simulink model "RGP_regression_th"  (R2018b)
settings: Solver=FixedStepAuto  StartTime=0.0  StopTime=timeVec(end)  FixedStep=(timeVec(2)-timeVec(1))  RelTol=1e-3
values from neighbouring files (symbols this model uses):
  postVarCtrlGain = 1    [RGP_regression_ts.m]
libraries: simulink x2, RGP_ctrl x1, RGP_regression x1
settings Model: Creator=asiddiq2  LastModifiedBy=Ayaz
settings DataIOCC: ReturnWorkspaceOutputs=on

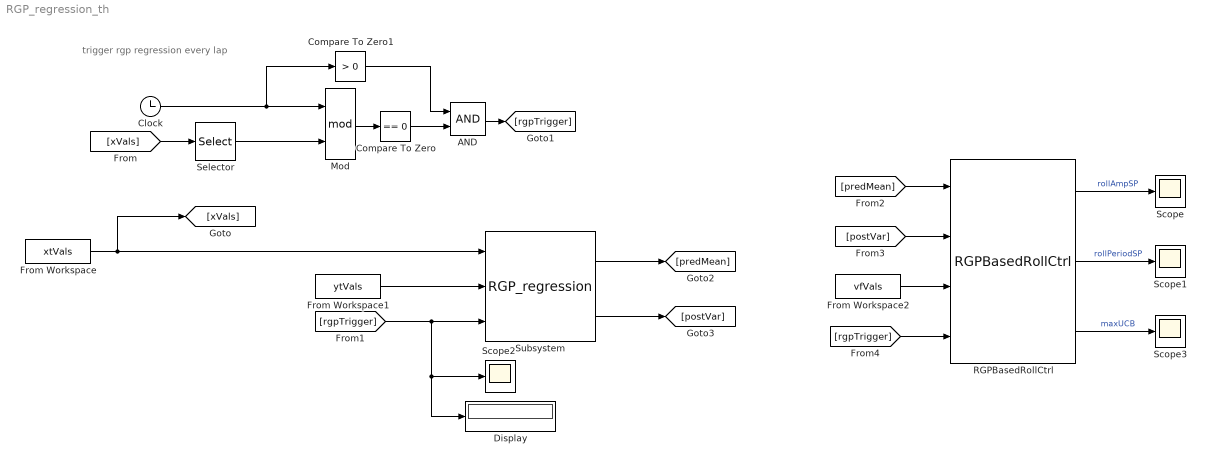
== system RGP_regression_th ==
  note: trigger rgp regression every lap
  AND : Logic  AllPortsSameDT=off  OutDataTypeStr=boolean
  Clock : Clock
  Compare To Zero : simulink/Logic and Bit Operations/Compare To Zero  relop===  OutDataTypeStr=boolean
  Compare To Zero1 : simulink/Logic and Bit Operations/Compare To Zero  relop=>  OutDataTypeStr=boolean
  Display : Display
  From Workspace : FromWorkspace  VariableName=xtVals
  From Workspace1 : FromWorkspace  VariableName=ytVals
  From Workspace2 : FromWorkspace  VariableName=vfVals
  Mod : Math  Operator=mod  SaturateOnIntegerOverflow=on
  RGPBasedRollCtrl : RGP_ctrl/RGPBasedRollCtrl  predMeanGain=predMeanCtrlGain  postVarGain=2^postVarCtrlGain  xBasis=basisVector  initRollAmpDeg=0  initRollPeriodSec=20
  Scope{,1..3} (4 alike) : Scope
  Selector : Selector  InputPortWidth=3  IndexOptions=Index vector (dialog)  Indices=2  OutputSizes=1
  Subsystem : RGP_regression/RGP_regression  xBasis=basisVector  meanFcnProp=meanFcnProperties  meanFcnVec=meanFcnVector  hyperParams=hyperParameters  basisCovMat=basisCovMat  noiseVar=noiseVariance
  wires:
  From Workspace1/1 -> Subsystem/2
  [rgpTrigger] -> Display/1, Scope2/1, Subsystem/3
  Subsystem/1 -> [predMean]
  Subsystem/2 -> [postVar]
  From Workspace/1 -> [xVals], Subsystem/1
  Clock/1 -> Compare To Zero1/1, Mod/1
  Selector/1 -> Mod/2
  Mod/1 -> Compare To Zero/1
  [xVals] -> Selector/1
  Compare To Zero/1 -> AND/2
  Compare To Zero1/1 -> AND/1
  AND/1 -> [rgpTrigger]
  [predMean] -> RGPBasedRollCtrl/1
  [postVar] -> RGPBasedRollCtrl/2
  From Workspace2/1 -> RGPBasedRollCtrl/3
  [rgpTrigger] -> RGPBasedRollCtrl/4
  RGPBasedRollCtrl/1 -> Scope/1  "rollAmpSP"
  RGPBasedRollCtrl/2 -> Scope1/1  "rollPeriodSP"
  RGPBasedRollCtrl/3 -> Scope3/1  "maxUCB"
